simulink model "ejer2_1"  (R2022b)
settings: Solver=VariableStepAuto  StartTime=0.0  StopTime=10.0  RelTol=1e-3
InitFcn:
  | pd1 = -4;
  | pd2 =-4;
  | k=0.5;
  | b=1;
  | m=1;
  | A = [0,1;-k/m, -b/m];
  | B = [0;1/m];
  | eigs(A);
  | Mc = [B, A*B];A = [0,1;-k/m, -b/m];
  | C = eye(2);
  | H = (A-pd1*eye(2))*(A-pd2*eye(2));
  | K = -[0,1]*(inv(Mc)*H);
settings Model: Creator=garci  LastModifiedBy=garci

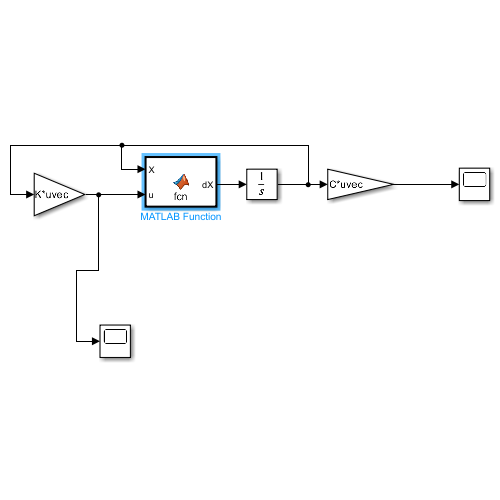
[thumbnail: Simulink's stored preview of the top-level diagram]
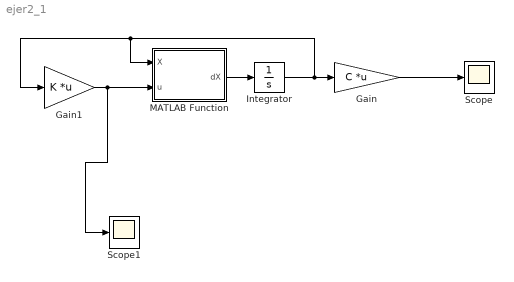
== system ejer2_1 ==
  Gain : Gain  Gain=C  Multiplication=Matrix(K*u) (u vector)
  Gain1 : Gain  Gain=K  Multiplication=Matrix(K*u) (u vector)
  Integrator : Integrator
  MATLAB Function : MATLAB Function  TreatAsAtomicUnit=on
  Scope : Scope
  Scope1 : Scope
  wires:
  MATLAB Function/1(dX) -> Integrator/1
  Integrator/1 -> Gain1/1, MATLAB Function/1(X), Gain/1
  Gain/1 -> Scope/1
  Gain1/1 -> Scope1/1, MATLAB Function/2(u)

== matlab function ejer2_1/MATLAB Function ==
  data: X input; u input; dX output; A parameter; B parameter
function dX = fcn(X,u, A, B)

dX = A*X +B*u;
